simulink model "f14"  (Simulink 7.6)
settings: Solver=ode45  SolverMode=SingleTasking  StartTime=0.0  StopTime=60  RelTol=1e-4  AbsTol=1e-6
PreLoadFcn:
  | f14dat
values from neighbouring files (symbols this model uses):
  a = 2.5348    [f14_digital_data.mat]    (also in f14dat_digital.m; sanim.m = size(vert); sanim3dof.m = size(vert))
  b = 64.13    [f14_digital_data.mat]    (also in f14dat_digital.m)
  g = 9.81    [aero_guid_dat.m]    (also in f14_digital_data.mat = 32.2; f14dat_digital.m = 32.2)
  Ka = 0.677    [f14_digital_data.mat]    (also in f14dat_digital.m)
  Kf = -1.746    [f14_digital_data.mat]    (also in f14dat_digital.m)
  Ki = -3.864    [f14_digital_data.mat]    (also in f14dat_digital.m)
  Kq = 0.8156    [f14_digital_data.mat]    (also in f14dat_digital.m)
  Md = -6.8847    [f14_digital_data.mat]    (also in f14dat_digital.m)
  Mq = -0.6571    [f14_digital_data.mat]    (also in f14dat_digital.m)
  Mw = -0.00592    [f14_digital_data.mat]    (also in f14dat_digital.m)
  Swg = 3    [f14_digital_data.mat]    (also in f14dat_digital.m)
  Ta = 0.05    [f14_digital_data.mat]    (also in f14dat_digital.m)
  Tal = 0.3959    [f14_digital_data.mat]    (also in f14dat_digital.m)
  Ts = 0.1    [f14_digital_data.mat]    (also in f14dat_digital.m)
  Uo = 689.4    [f14_digital_data.mat]    (also in f14dat_digital.m)
  Vto = 690.4    [f14_digital_data.mat]    (also in f14dat_digital.m)
  W1 = 2.971    [f14_digital_data.mat]    (also in f14dat_digital.m)
  W2 = 4.144    [f14_digital_data.mat]    (also in f14dat_digital.m)
  Zd = -63.9979    [f14_digital_data.mat]    (also in f14dat_digital.m)
  Zw = -0.6385    [f14_digital_data.mat]    (also in f14dat_digital.m)
libraries: simulink3 x1
settings Model: Creator=The MathWorks Inc.  ExtModeTrigMode=oneshot  ExtModeArmWhenConnect=off  ExtModeAutoUpdateStatusClock=off
settings DataIOCC: ExternalInput=[]  InitialState=[]  LimitDataPoints=off  SaveOutput=off  SaveTime=off
settings OptimizationCC: BlockReduction=off  BooleanDataType=off  InitFltsAndDblsToZero=on
settings DebuggingCC: SaveWithParameterizedLinksMsg=none  SignalResolutionControl=TryResolveAllWithWarning  SolverPrmCheckMsg=none  MultiTaskDSMMsg=warning  MultiTaskCondExecSysMsg=none  IntegerOverflowMsg=none
settings RTWCC: IncludeERTFirstTime=on
settings CodeAppCC: CustomSymbolStrFcn=$F$N$M
settings GRTTargetCC: TargetFcnLib=ansi_tfl_tmw.mat

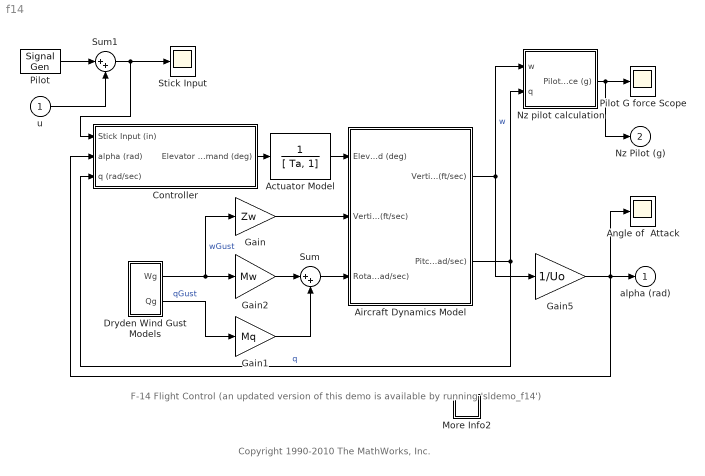
== system f14 ==
  note: F-14 Flight Control
      | (an updated version of this demo is available
      | by running 'sldemo_f14')
  note: Copyright 1990-2010 The MathWorks, Inc.
  u : Inport
  Actuator Model : TransferFcn  Denominator=[ Ta, 1]
  Aircraft Dynamics Model : Subsystem
  Angle of  Attack : Scope
      settings: TickLabels=on  TimeRange=60  YMin=-1.25  YMax=1.25  DataFormat=Array
  Controller : Subsystem
  Dryden Wind Gust Models : Subsystem
  Gain : Gain  Gain=Zw  SaturateOnIntegerOverflow=on  OutDataTypeStr=Inherit: Same as input  ParamDataTypeStr=Inherit: Same as input
  Gain1 : Gain  Gain=Mq  SaturateOnIntegerOverflow=on  OutDataTypeStr=Inherit: Same as input  ParamDataTypeStr=Inherit: Same as input
  Gain2 : Gain  Gain=Mw  SaturateOnIntegerOverflow=on  OutDataTypeStr=Inherit: Same as input  ParamDataTypeStr=Inherit: Same as input
  Gain5 : Gain  Gain=1/Uo  SaturateOnIntegerOverflow=on  OutDataTypeStr=Inherit: Same as input  ParamDataTypeStr=Inherit: Same as input
  More Info2 : Subsystem
      settings: OpenFcn=showdemo('sldemo_f14')
      mask Display: disp('?')
  Nz pilot calculation : Subsystem
  Pilot : SignalGenerator  WaveForm=square  Frequency=0.500000  Units=rad/sec
  Pilot G force Scope : Scope
      settings: TickLabels=on  TimeRange=60  YMin=-15  YMax=15  DataFormat=Array
  Stick Input : Scope
      settings: TickLabels=on  TimeRange=60  YMin=-1.5  YMax=1.5  DataFormat=Array
  Sum : Sum  Inputs=|++  SaturateOnIntegerOverflow=on  InputSameDT=on  OutDataTypeStr=Inherit: Same as first input
  Sum1 : Sum  Inputs=|++  SaturateOnIntegerOverflow=on  InputSameDT=on  OutDataTypeStr=Inherit: Same as first input
  alpha (rad) : Outport  InitialOutput=0
  Nz Pilot (g) : Outport  Port=2  InitialOutput=0
  wires:
  Gain5/1 -> alpha (rad)/1, Angle of  Attack/1, Controller/2(alpha (rad))
  Aircraft Dynamics Model/1(Vertical Velocity w (ft/sec)) -> Gain5/1, Nz pilot calculation/1(w)  "w"
  Nz pilot calculation/1(Pilot g force (g)) -> Pilot G force Scope/1, Nz Pilot (g)/1
  Gain2/1 -> Sum/1
  Gain/1 -> Aircraft Dynamics Model/2(Vertical Gust wGust (ft/sec))
  Pilot/1 -> Sum1/1
  u/1 -> Sum1/2
  Dryden Wind Gust Models/2(Qg) -> Gain1/1  "qGust"
  Dryden Wind Gust Models/1(Wg) -> Gain2/1, Gain/1  "wGust"
  Sum/1 -> Aircraft Dynamics Model/3(Rotary Gust qGust (rad/sec))
  Gain1/1 -> Sum/2
  Aircraft Dynamics Model/2(Pitch Rate q (rad/sec)) -> Nz pilot calculation/2(q), Controller/3(q (rad/sec))  "q"
  Actuator Model/1 -> Aircraft Dynamics Model/1(Elevator Deflection d (deg))
  Controller/1(Elevator Command (deg)) -> Actuator Model/1
  Sum1/1 -> Stick Input/1, Controller/1(Stick Input (in))

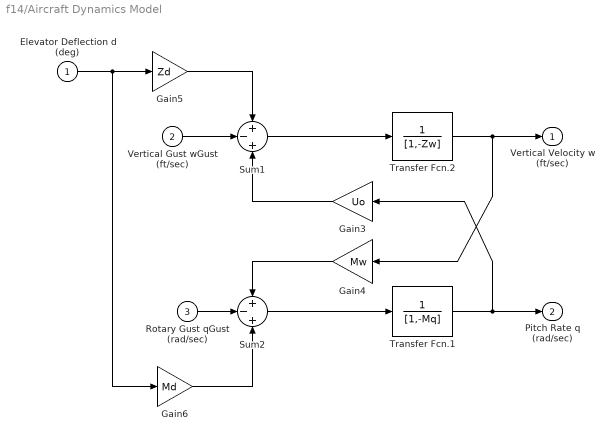
== system f14/Aircraft Dynamics Model ==
  Elevator Deflection d (deg) : Inport
  Vertical Gust wGust (ft/sec) : Inport  Port=2
  Rotary Gust qGust (rad/sec) : Inport  Port=3
  Gain3 : Gain  Gain=Uo  SaturateOnIntegerOverflow=on  OutDataTypeStr=Inherit: Same as input  ParamDataTypeStr=Inherit: Same as input
  Gain4 : Gain  Gain=Mw  SaturateOnIntegerOverflow=on  OutDataTypeStr=Inherit: Same as input  ParamDataTypeStr=Inherit: Same as input
  Gain5 : Gain  Gain=Zd  SaturateOnIntegerOverflow=on  OutDataTypeStr=Inherit: Same as input  ParamDataTypeStr=Inherit: Same as input
  Gain6 : Gain  Gain=Md  SaturateOnIntegerOverflow=on  OutDataTypeStr=Inherit: Same as input  ParamDataTypeStr=Inherit: Same as input
  Sum1 : Sum  Inputs=+-+  SaturateOnIntegerOverflow=on  InputSameDT=on  OutDataTypeStr=Inherit: Same as first input
  Sum2 : Sum  Inputs=+-+  SaturateOnIntegerOverflow=on  InputSameDT=on  OutDataTypeStr=Inherit: Same as first input
  Transfer Fcn.1 : TransferFcn  Denominator=[1,-Mq]
  Transfer Fcn.2 : TransferFcn  Denominator=[1,-Zw]
  Vertical Velocity w (ft/sec) : Outport  InitialOutput=0
  Pitch Rate q (rad/sec) : Outport  Port=2  InitialOutput=0
  wires:
  Transfer Fcn.2/1 -> Vertical Velocity w (ft/sec)/1, Gain4/1
  Transfer Fcn.1/1 -> Pitch Rate q (rad/sec)/1, Gain3/1
  Gain6/1 -> Sum2/3
  Gain5/1 -> Sum1/1
  Gain3/1 -> Sum1/3
  Rotary Gust qGust (rad/sec)/1 -> Sum2/2
  Sum2/1 -> Transfer Fcn.1/1
  Sum1/1 -> Transfer Fcn.2/1
  Gain4/1 -> Sum2/1
  Vertical Gust wGust (ft/sec)/1 -> Sum1/2
  Elevator Deflection d (deg)/1 -> Gain5/1, Gain6/1

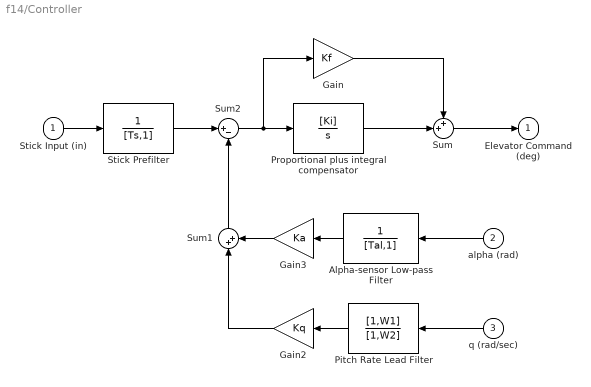
== system f14/Controller ==
  Stick Input (in) : Inport
  alpha (rad) : Inport  Port=2
  q (rad/sec) : Inport  Port=3
  Alpha-sensor Low-pass Filter : TransferFcn  Denominator=[Tal,1]
  Gain : Gain  Gain=Kf  SaturateOnIntegerOverflow=on  OutDataTypeStr=Inherit: Same as input  ParamDataTypeStr=Inherit: Same as input
  Gain2 : Gain  Gain=Kq  SaturateOnIntegerOverflow=on  OutDataTypeStr=Inherit: Same as input  ParamDataTypeStr=Inherit: Same as input
  Gain3 : Gain  Gain=Ka  SaturateOnIntegerOverflow=on  OutDataTypeStr=Inherit: Same as input  ParamDataTypeStr=Inherit: Same as input
  Pitch Rate Lead Filter : TransferFcn  Numerator=[1,W1]  Denominator=[1,W2]
  Proportional plus integral compensator : TransferFcn  Numerator=[Ki]  Denominator=[1,0]
  Stick Prefilter : TransferFcn  Denominator=[Ts,1]
  Sum : Sum  Inputs=++|  SaturateOnIntegerOverflow=on  InputSameDT=on  OutDataTypeStr=Inherit: Same as first input
  Sum1 : Sum  Inputs=|++  SaturateOnIntegerOverflow=on  InputSameDT=on  OutDataTypeStr=Inherit: Same as first input
  Sum2 : Sum  Inputs=|+-  SaturateOnIntegerOverflow=on  InputSameDT=on  OutDataTypeStr=Inherit: Same as first input
  Elevator Command (deg) : Outport  InitialOutput=0
  wires:
  Sum2/1 -> Proportional plus integral compensator/1, Gain/1
  Gain/1 -> Sum/1
  Proportional plus integral compensator/1 -> Sum/2
  Stick Prefilter/1 -> Sum2/1
  Sum/1 -> Elevator Command (deg)/1
  Gain2/1 -> Sum1/1
  Gain3/1 -> Sum1/2
  Sum1/1 -> Sum2/2
  Pitch Rate Lead Filter/1 -> Gain2/1
  q (rad/sec)/1 -> Pitch Rate Lead Filter/1
  Alpha-sensor Low-pass Filter/1 -> Gain3/1
  alpha (rad)/1 -> Alpha-sensor Low-pass Filter/1
  Stick Input (in)/1 -> Stick Prefilter/1

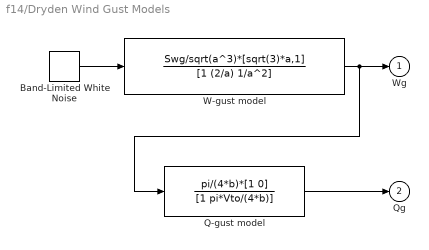
== system f14/Dryden Wind Gust Models ==
  Band-Limited White Noise : simulink3/Sources/Band-Limited White Noise  Cov=1  Ts=0.1  seed=[23341]
  Q-gust model : TransferFcn  Numerator=pi/(4*b)*[1 0]  Denominator=[1 pi*Vto/(4*b)]
  W-gust model : TransferFcn  Numerator=Swg/sqrt(a^3)*[sqrt(3)*a,1]  Denominator=[1 (2/a) 1/a^2]
  Wg : Outport  InitialOutput=0
  Qg : Outport  Port=2  InitialOutput=0
  wires:
  Band-Limited White Noise/1 -> W-gust model/1
  Q-gust model/1 -> Qg/1
  W-gust model/1 -> Wg/1, Q-gust model/1

== system f14/More Info2 ==

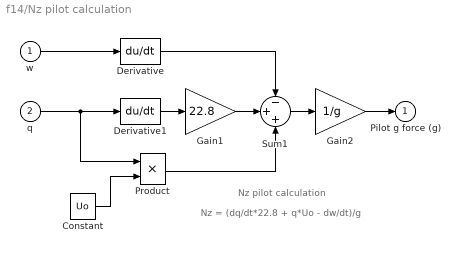
== system f14/Nz pilot calculation ==
  note: Nz pilot calculation
  note: Nz = (dq/dt*22.8 + q*Uo - dw/dt)/g
  w : Inport
  q : Inport  Port=2
  Constant : Constant  Value=Uo
  Derivative : Derivative
  Derivative1 : Derivative
  Gain1 : Gain  Gain=22.8  SaturateOnIntegerOverflow=on  OutDataTypeStr=Inherit: Same as input  ParamDataTypeStr=Inherit: Same as input
  Gain2 : Gain  Gain=1/g  SaturateOnIntegerOverflow=on  OutDataTypeStr=Inherit: Same as input  ParamDataTypeStr=Inherit: Same as input
  Product : Product  SaturateOnIntegerOverflow=on  RndMeth=Zero  InputSameDT=on  OutDataTypeStr=Inherit: Same as first input
  Sum1 : Sum  Inputs=-++  SaturateOnIntegerOverflow=on  InputSameDT=on  OutDataTypeStr=Inherit: Same as first input
  Pilot g force (g) : Outport  InitialOutput=0
  wires:
  q/1 -> Product/1, Derivative1/1
  Constant/1 -> Product/2
  Gain2/1 -> Pilot g force (g)/1
  Sum1/1 -> Gain2/1
  Derivative1/1 -> Gain1/1
  Gain1/1 -> Sum1/2
  Product/1 -> Sum1/3
  Derivative/1 -> Sum1/1
  w/1 -> Derivative/1
